simulink model "Validate"  (R2024b)
settings: Solver=VariableStepAuto  StartTime=0.0  StopTime=1  RelTol=1e-3
InitFcn:
  | clc;
  | clear;
  | 
  | Vdc = 100;
  | 
  | R1 = 1e-3;
  | L1 = -0.0084;
  | Lm = 3.5483e-4;
  | 
  | R2 = 1e-3;
  | L2 = 0.0189;
  | n2 = 0.2337;
  | 
  | R3 = 1e-3;
  | L3 = 0.0191;
  | n3 = 0.2242;
libraries: spsVoltageMeasurementLib x5, spsCurrentMeasurementLib x4, spsLinearTransformerLib x4, spsSeriesRLCBranchLib x4, spsDCVoltageSourceLib x3, spsFullBridgeConverterLib x3, spsGroundLib x3, spsSawtoothGeneratorLib x2, sps_lib x1
settings Model: Creator=wang.shum  LastModifiedBy=wang.shum

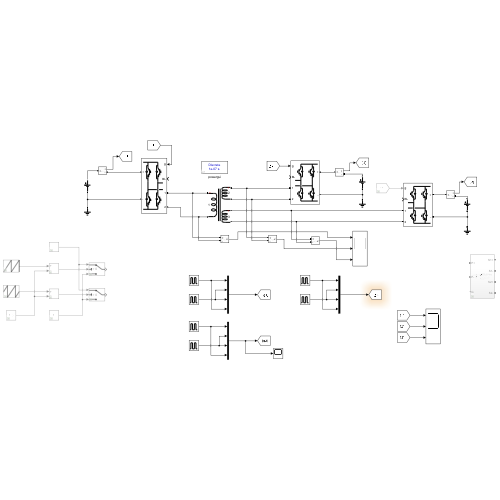
[thumbnail: Simulink's stored preview of the top-level diagram]
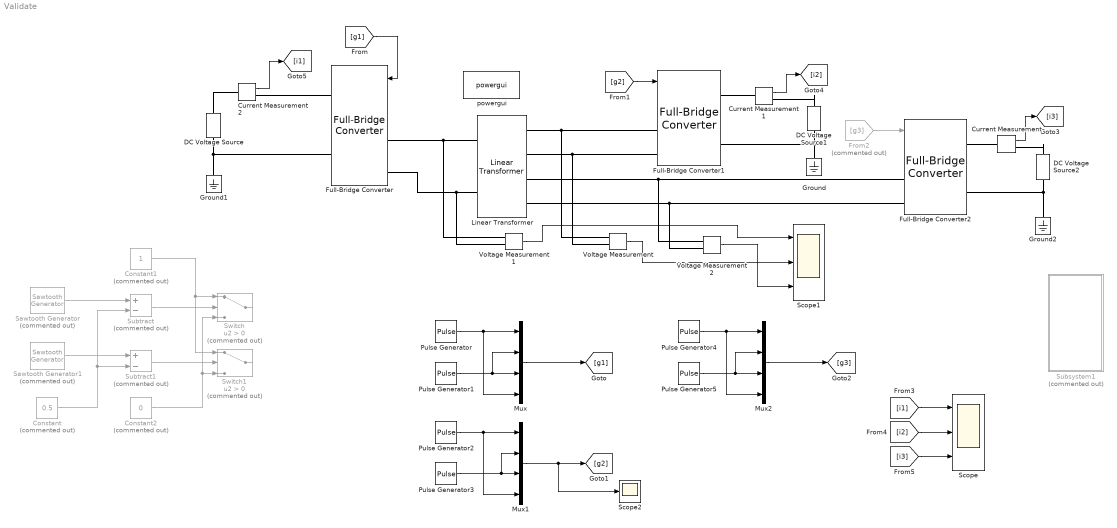
== system Validate ==
  Constant : Constant  Commented=on  Value=0.5
  Constant1 : Constant  Commented=on
  Constant2 : Constant  Commented=on  Value=0
  Current Measurement : spsCurrentMeasurementLib/Current Measurement  PhasorSimulation=off  OutputType=Complex  PSBequivalent=0
  Current Measurement1 : spsCurrentMeasurementLib/Current Measurement  PhasorSimulation=off  OutputType=Complex  PSBequivalent=0
  Current Measurement2 : spsCurrentMeasurementLib/Current Measurement  PhasorSimulation=off  OutputType=Complex  PSBequivalent=0
  DC Voltage Source : spsDCVoltageSourceLib/DC Voltage Source  Amplitude=Vdc  Measurements=None
  DC Voltage Source1 : spsDCVoltageSourceLib/DC Voltage Source  Amplitude=Vdc  Measurements=None
  DC Voltage Source2 : spsDCVoltageSourceLib/DC Voltage Source  Amplitude=Vdc  Measurements=None
  From2 : From  Commented=on  GotoTag=g3
  Full-Bridge Converter : spsFullBridgeConverterLib/Full-Bridge Converter  ModelType=Switching devices  Ron=1e-3  Rs=1e6  Cs=inf  Vforward=[0,0]  Ron_Diode=1e-3  Rs_Diode=1e6  Cs_Diode=inf  Vf_Diode=1e-3  Rs_CurrentSource=inf  Ron_ACsource=1e-3
      settings: LibrarySourceBlock=sps_lib/Power Electronics/Full-Bridge Converter
  Full-Bridge Converter1 : spsFullBridgeConverterLib/Full-Bridge Converter  ModelType=Switching devices  Ron=1e-3  Rs=1e6  Cs=inf  Vforward=[0,0]  Ron_Diode=1e-3  Rs_Diode=1e6  Cs_Diode=inf  Vf_Diode=1e-3  Rs_CurrentSource=inf  Ron_ACsource=1e-3
      settings: LibrarySourceBlock=sps_lib/Power Electronics/Full-Bridge Converter
  Full-Bridge Converter2 : spsFullBridgeConverterLib/Full-Bridge Converter  ModelType=Switching devices  Ron=1e-3  Rs=1e6  Cs=inf  Vforward=[0,0]  Ron_Diode=1e-3  Rs_Diode=1e6  Cs_Diode=inf  Vf_Diode=1e-3  Rs_CurrentSource=inf  Ron_ACsource=1e-3
      settings: LibrarySourceBlock=sps_lib/Power Electronics/Full-Bridge Converter
  Ground : spsGroundLib/Ground  LConnTagsString=a
  Ground1 : spsGroundLib/Ground  LConnTagsString=a
  Ground2 : spsGroundLib/Ground  LConnTagsString=a
  Linear Transformer : spsLinearTransformerLib/Linear Transformer  UNITS=SI  NominalPower=[ 1e3 1e5 ]  winding1=[100 1e-3 L1]  winding2=[100*n2 1e-3 L2]  ThreeWindings=on  winding3=[100*n3 1e-3 L3]  RmLm=[1e-3 Lm]  Measurements=None  DataType=on
  Mux : Mux
  Mux1 : Mux
  Mux2 : Mux
  Pulse Generator : DiscretePulseGenerator  PulseType=Time based  Period=1e-5  PulseWidth=50
  Pulse Generator1 : DiscretePulseGenerator  PulseType=Time based  Period=1e-5  PulseWidth=50  PhaseDelay=0.5e-5
  Pulse Generator2 : DiscretePulseGenerator  PulseType=Time based  Period=1e-5  PulseWidth=50  PhaseDelay=0.2e-5
  Pulse Generator3 : DiscretePulseGenerator  PulseType=Time based  Period=1e-5  PulseWidth=50  PhaseDelay=0.7e-5
  Pulse Generator4 : DiscretePulseGenerator  PulseType=Time based  Period=1e-5  PulseWidth=50
  Pulse Generator5 : DiscretePulseGenerator  PulseType=Time based  Period=1e-5  PulseWidth=50  PhaseDelay=0.5e-5
  Sawtooth Generator : spsSawtoothGeneratorLib/Sawtooth Generator  Commented=on  Freq=1e5  Phase=0  Ts=0
  Sawtooth Generator1 : spsSawtoothGeneratorLib/Sawtooth Generator  Commented=on  Freq=1e5  Phase=180  Ts=0
  Scope : Scope  NumInputPorts=3
  Scope1 : Scope  NumInputPorts=3
  Scope2 : Scope
  Subsystem1 : Subsystem  Commented=on
  Subtract : Sum  Commented=on  Inputs=+-
  Subtract1 : Sum  Commented=on  Inputs=+-
  Switch : Switch  Commented=on  Criteria=u2 > Threshold  SaturateOnIntegerOverflow=off  InputSameDT=off
  Switch1 : Switch  Commented=on  Criteria=u2 > Threshold  SaturateOnIntegerOverflow=off  InputSameDT=off
  Voltage Measurement : spsVoltageMeasurementLib/Voltage Measurement  PhasorSimulation=off  OutputType=Complex  PSBequivalent=0
  Voltage Measurement1 : spsVoltageMeasurementLib/Voltage Measurement  PhasorSimulation=off  OutputType=Complex  PSBequivalent=0
  Voltage Measurement2 : spsVoltageMeasurementLib/Voltage Measurement  PhasorSimulation=off  OutputType=Complex  PSBequivalent=0
  powergui : sps_lib/powergui  Priority=1  SimulationMode=Discrete  SampleTime=1e-7  frequency=60  Iterations=50  frequencyindice=0  Pbase=100e6  ErrMax=1e-4  UnitsV=kV  UnitsW=MW  buscounter=0  FunctionMessages=off  echomessages=off  EnableUseOfTLC=off  CurrentSourceSwitches=off  DisableSnubberDevices=off  DisableRonSwitches=off  DisableVfSwitches=off  DisplayEquations=off  AutomaticDiscreteSolvers=off  SolverType=Tustin/Backward Euler (TBE)  Interpol=off  ExternalGateDelay=off  methode=off  Ts=100  x0status=blocks  SPID=on  SwTol=0  HookPort=off  NonlinearTolerance=1e-4  nMaxIteration=100  ContinueOnMaxIteration=off  RestoreLinks=warning  ResistiveCurrentMeasurement=off  Frange=[0:2:500]  Ylog=off  Xlog=on  ShowGrid=off  save=off  variable=ZData  structure=0  ZoomFFT=off  StartTime=0.0  cycles=1  DisplayStyle=1  fundamental=60  FreqAxis=off  MaxFrequency=1000  frequencyindicesteady=1  RmsSteady=1  display=off
  wires:
  Sawtooth Generator/1 -> Subtract/1
  Constant/1 -> Subtract1/2, Subtract/2
  Sawtooth Generator1/1 -> Subtract1/1
  Subtract/1 -> Switch/2
  Constant1/1 -> Switch1/1, Switch/1
  Subtract1/1 -> Switch1/2
  Constant2/1 -> Switch/3, Switch1/3
  Pulse Generator/1 -> Mux/4, Mux/1
  Pulse Generator1/1 -> Mux/2, Mux/3
  Mux/1 -> [g1]
  [g1] -> Full-Bridge Converter/1
  Mux1/1 -> Scope2/1, [g2]
  Pulse Generator4/1 -> Mux2/4, Mux2/1
  Pulse Generator5/1 -> Mux2/2, Mux2/3
  Mux2/1 -> [g3]
  [g2] -> Full-Bridge Converter1/1
  From2/1 -> Full-Bridge Converter2/1
  Current Measurement/1 -> [i3]
  Current Measurement1/1 -> [i2]
  Current Measurement2/1 -> [i1]
  [i1] -> Scope/1
  [i2] -> Scope/2
  [i3] -> Scope/3
  Voltage Measurement1/1 -> Scope1/1
  Voltage Measurement/1 -> Scope1/2
  Voltage Measurement2/1 -> Scope1/3
  Pulse Generator2/1 -> Mux1/4, Mux1/1
  Pulse Generator3/1 -> Mux1/3, Mux1/2
  connections:
  Linear Transformer/LConn2 -- Voltage Measurement1/LConn2 -- Full-Bridge Converter/LConn2
  Linear Transformer/LConn1 -- Voltage Measurement1/LConn1 -- Full-Bridge Converter/LConn1
  Linear Transformer/RConn2 -- Voltage Measurement/LConn2 -- Full-Bridge Converter1/LConn2
  Linear Transformer/RConn1 -- Voltage Measurement/LConn1 -- Full-Bridge Converter1/LConn1
  Linear Transformer/RConn3 -- Voltage Measurement2/LConn1 -- Full-Bridge Converter2/LConn1
  Full-Bridge Converter2/LConn2 -- Voltage Measurement2/LConn2 -- Linear Transformer/RConn4
  DC Voltage Source/LConn1 -- Ground1/LConn1 -- Full-Bridge Converter/RConn2
  DC Voltage Source1/LConn1 -- Full-Bridge Converter1/RConn2 -- Ground/LConn1
  Full-Bridge Converter2/RConn2 -- Ground2/LConn1 -- DC Voltage Source2/LConn1
  Current Measurement/LConn1 -- Full-Bridge Converter2/RConn1
  DC Voltage Source2/RConn1 -- Current Measurement/RConn1
  Current Measurement1/LConn1 -- Full-Bridge Converter1/RConn1
  DC Voltage Source1/RConn1 -- Current Measurement1/RConn1
  Current Measurement2/RConn1 -- Full-Bridge Converter/RConn1
  Current Measurement2/LConn1 -- DC Voltage Source/RConn1

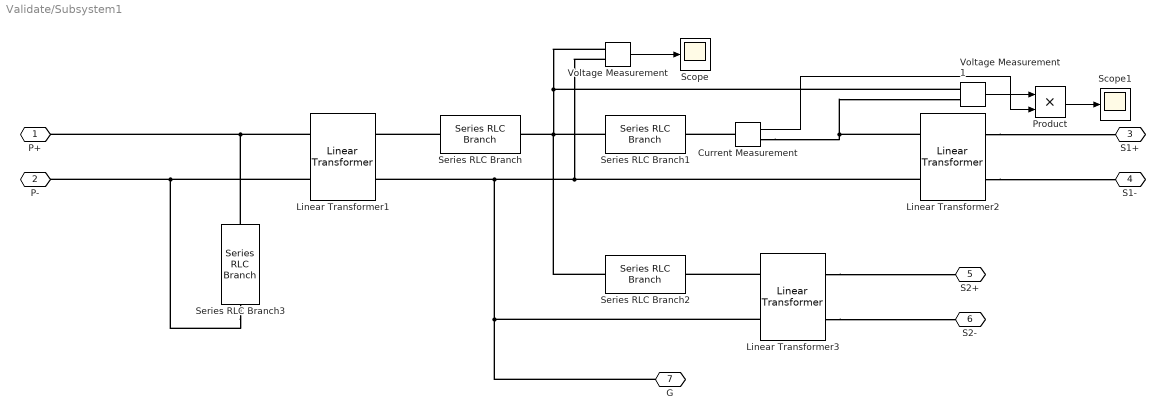
== system Validate/Subsystem1 ==
  Current Measurement : spsCurrentMeasurementLib/Current Measurement  PhasorSimulation=off  OutputType=Complex  PSBequivalent=0
  Linear Transformer1 : spsLinearTransformerLib/Linear Transformer  UNITS=SI  NominalPower=[1e3 1e5 ]  winding1=[100 1e-3 1e-9]  winding2=[100 1e-3 1e-9]  ThreeWindings=off  winding3=[3.15e+05 1.9845e+05 12.634]  RmLm=[5000 5]  Measurements=None  DataType=on
  Linear Transformer2 : spsLinearTransformerLib/Linear Transformer  UNITS=SI  NominalPower=[1e3 1e5 ]  winding1=[100 1e-3 1e-9]  winding2=[100*n2 1e-3 1e-9]  ThreeWindings=off  winding3=[3.15e+05 1.9845e+05 12.634]  RmLm=[5000 5]  Measurements=None  DataType=on
  Linear Transformer3 : spsLinearTransformerLib/Linear Transformer  UNITS=SI  NominalPower=[1e3 1e5 ]  winding1=[100 1e-3 1e-9]  winding2=[100*n3 1e-3 1e-9]  ThreeWindings=off  winding3=[3.15e+05 1.9845e+05 12.634]  RmLm=[5000 5]  Measurements=None  DataType=on
  Product : Product
  Scope : Scope
  Scope1 : Scope
  Series RLC Branch : spsSeriesRLCBranchLib/Series RLC Branch  LConnTagsString=__new0  RConnTagsString=__new0  BranchType=RL  Resistance=R1  Inductance=L1  SetiL0=off  InitialCurrent=0  Capacitance=1e-6  Setx0=off  InitialVoltage=0  Measurements=None
  Series RLC Branch1 : spsSeriesRLCBranchLib/Series RLC Branch  LConnTagsString=__new0  RConnTagsString=__new0  BranchType=RL  Resistance=R2  Inductance=L2  SetiL0=off  InitialCurrent=0  Capacitance=1e-6  Setx0=off  InitialVoltage=0  Measurements=None
  Series RLC Branch2 : spsSeriesRLCBranchLib/Series RLC Branch  LConnTagsString=__new0  RConnTagsString=__new0  BranchType=RL  Resistance=R3  Inductance=L3  SetiL0=off  InitialCurrent=0  Capacitance=1e-6  Setx0=off  InitialVoltage=0  Measurements=None
  Series RLC Branch3 : spsSeriesRLCBranchLib/Series RLC Branch  LConnTagsString=__new0  RConnTagsString=__new0  BranchType=RL  Resistance=R1  Inductance=Lm  SetiL0=off  InitialCurrent=0  Capacitance=1e-6  Setx0=off  InitialVoltage=0  Measurements=None
  Voltage Measurement : spsVoltageMeasurementLib/Voltage Measurement  PhasorSimulation=off  OutputType=Complex  PSBequivalent=0
  Voltage Measurement1 : spsVoltageMeasurementLib/Voltage Measurement  PhasorSimulation=off  OutputType=Complex  PSBequivalent=0
  P+ : PMIOPort  Side=Left
  P- : PMIOPort  Port=2  Side=Left
  S1+ : PMIOPort  Port=3  Side=Right
  S1- : PMIOPort  Port=4  Side=Right
  S2+ : PMIOPort  Port=5  Side=Right
  S2- : PMIOPort  Port=6  Side=Right
  G : PMIOPort  Port=7  Side=Left
  wires:
  Product/1 -> Scope1/1
  Current Measurement/1 -> Product/2
  Voltage Measurement1/1 -> Product/1
  Voltage Measurement/1 -> Scope/1
  connections:
  Current Measurement/LConn1 -- Series RLC Branch1/RConn1
  Voltage Measurement/LConn2 -- Linear Transformer2/LConn2 -- Linear Transformer1/RConn2 -- G/RConn1 -- Linear Transformer3/LConn2
  Linear Transformer3/RConn2 -- S2-/RConn1
  Linear Transformer3/RConn1 -- S2+/RConn1
  Linear Transformer3/LConn1 -- Series RLC Branch2/RConn1
  Current Measurement/RConn1 -- Linear Transformer2/LConn1 -- Voltage Measurement1/LConn2
  Voltage Measurement/LConn1 -- Voltage Measurement1/LConn1 -- Series RLC Branch2/LConn1 -- Series RLC Branch1/LConn1 -- Series RLC Branch/RConn1
  Series RLC Branch/LConn1 -- Linear Transformer1/RConn1
  Series RLC Branch3/RConn1 -- Linear Transformer1/LConn2 -- P-/RConn1
  P+/RConn1 -- Linear Transformer1/LConn1 -- Series RLC Branch3/LConn1
  Linear Transformer2/RConn2 -- S1-/RConn1
  Linear Transformer2/RConn1 -- S1+/RConn1
